simulink model "SistemaPsk"  (R2017a)
settings: Solver=ode45  StartTime=0.0  StopTime=num_bits*tb  RelTol=1e-3
values from neighbouring files (symbols this model uses):
  Amplitud = sqrt(Potencia)    [Parametros_Sistema.m]
  ancho_filtro = rata_bit/2    (= 875)    [Parametros_Sistema.m]
  atenua_voltaje = sqrt(atenua_potencia)    [Parametros_Sistema.m]
  b = tb*0.2    (= 0.000114285714286)    [Parametros_Sistema.m]
  C = 1.5e-9    (= 1.5e-09)    [Parametros_Sistema.m]
  fc = 175e3    (= 175000)    [Parametros_Sistema.m]
  R1 = 200e3    (= 200000)    [Parametros_Sistema.m]
  R2 = 9e3    (= 9000)    [Parametros_Sistema.m]
  rata_bit = 1.75e3    (= 1750)    [Parametros_Sistema.m]
  retardo_canal = long/3e8    [Parametros_Sistema.m]
  retardo_decision = 1/rata_bit    (= 0.000571428571429)    [Parametros_Sistema.m]
  retardo_filtro = 1.7/rata_bit    (= 0.000971428571429)    [Parametros_Sistema.m]
  tb = 1/rb    (= 0.000571428571429)    [Codificacion.m]    (also in Parametros_Sistema.m)
libraries: dsparch4 x5, dspsigops x4, commsynccomp2 x2, powerlib_extras x2, commnoisgen2 x1, commrandsrc3 x1, simulink x1, simulink_extras x1
settings Model: Creator=PROYECTOS_101  LastModifiedBy=PROYECTOS_101

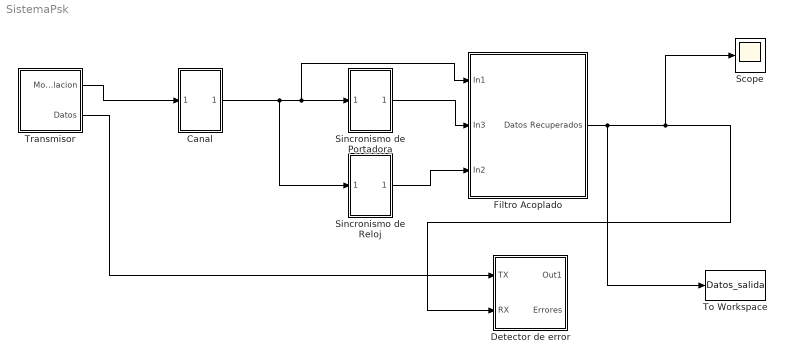
== system SistemaPsk ==
  Canal : Subsystem
  Detector de error : Subsystem
  "Filtro Acoplado " : Subsystem
  Scope : Scope
  Sincronismo de Portadora : Subsystem
  Sincronismo de Reloj : Subsystem
  To Workspace : ToWorkspace  VariableName=Datos_salida  SaveFormat=Structure With Time  SampleTime=-1
      settings: Save2DSignal=2-D array (concatenate along first dimension)
  "Transmisor " : Subsystem
  wires:
  Canal/1(Out1) -> Sincronismo de Reloj/1(In1), "Filtro Acoplado "/1(In1), Sincronismo de Portadora/1(In1)
  Sincronismo de Portadora/1(Out1) -> "Filtro Acoplado "/2(In3)
  Sincronismo de Reloj/1(Out1) -> "Filtro Acoplado "/3(In2)
  "Transmisor "/1(Modulacion) -> Canal/1(In1)
  "Transmisor "/2(Datos) -> Detector de error/1(TX)
  "Filtro Acoplado "/1(Datos Recuperados) -> To Workspace/1, Scope/1, Detector de error/2(RX)

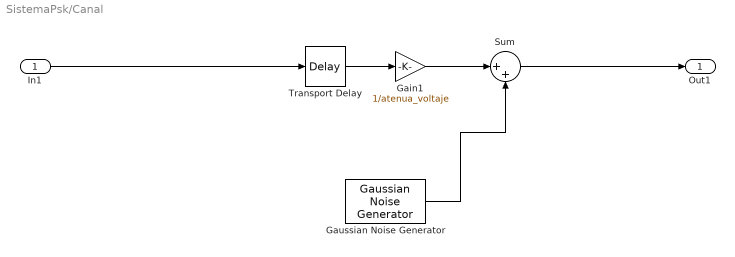
== system SistemaPsk/Canal ==
  In1 : Inport
  Gain1 : Gain  Gain=1/atenua_voltaje
  Gaussian Noise Generator : commnoisgen2/Gaussian Noise Generator  m=0  d=Potencia_ruido  s=61  Ts=1e-8  frameBased=off  sampPerFrame=1  orient=off  outDataType=double
  Sum : Sum  Inputs=|++
  Transport Delay : TransportDelay  DelayTime=retardo_canal
  Out1 : Outport
  wires:
  In1/1 -> Transport Delay/1
  Sum/1 -> Out1/1
  Gaussian Noise Generator/1 -> Sum/2
  Gain1/1 -> Sum/1
  Transport Delay/1 -> Gain1/1

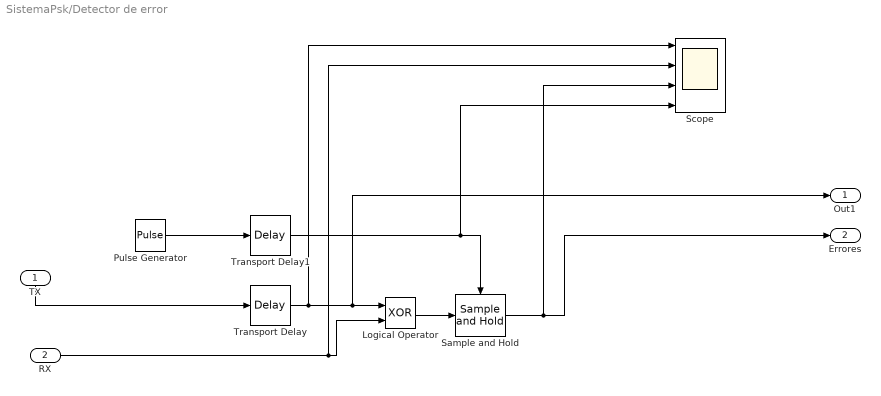
== system SistemaPsk/Detector de error ==
  TX : Inport
  RX : Inport  Port=2
  Logical Operator : Logic  Operator=XOR  AllPortsSameDT=off  OutDataTypeStr=boolean
  Pulse Generator : DiscretePulseGenerator  PulseType=Time based  Period=tb  PulseWidth=50
  Sample and Hold : dspsigops/Sample and Hold  trig=Rising edge  initCond=0  latchinput=off
  Scope : Scope  NumInputPorts=4
  Transport Delay : TransportDelay  DelayTime=retardo_canal+retardo_filtro+retardo_decision
  Transport Delay1 : TransportDelay  DelayTime=retardo_canal+retardo_filtro+retardo_decision
  Out1 : Outport
  Errores : Outport  Port=2
  wires:
  Transport Delay/1 -> Scope/1, Logical Operator/1, Out1/1
  Logical Operator/1 -> Sample and Hold/1
  Pulse Generator/1 -> Transport Delay1/1
  Transport Delay1/1 -> Scope/4, Sample and Hold/Trigger
  Sample and Hold/1 -> Scope/3, Errores/1
  TX/1 -> Transport Delay/1
  RX/1 -> Scope/2, Logical Operator/2

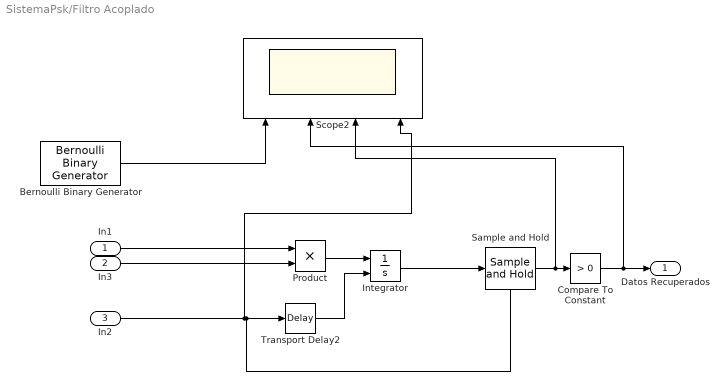
== system SistemaPsk/Filtro Acoplado  ==
  In1 : Inport
  In3 : Inport  Port=2
  In2 : Inport  Port=3
  Bernoulli Binary Generator : commrandsrc3/Bernoulli Binary Generator  ProbabilityOfZero=0.5  SeedSource=Parameter  Seed=61  SampleTime=tb  SamplesPerFrame=1  OutputDataType=double  SimulateUsing=Interpreted execution
  Compare To Constant : simulink/Logic and Bit Operations/Compare To Constant  relop=>  const=0  OutDataTypeStr=boolean
  Integrator : Integrator  ExternalReset=rising
  Product : Product
  Sample and Hold : dspsigops/Sample and Hold  trig=Rising edge  initCond=0  latchinput=off
  Scope2 : Scope  NumInputPorts=4
  Transport Delay2 : TransportDelay  DelayTime=1e-6
  Datos Recuperados : Outport
  wires:
  Integrator/1 -> Sample and Hold/1
  In1/1 -> Product/1
  Sample and Hold/1 -> Scope2/3, Compare To Constant/1
  Product/1 -> Integrator/1
  In2/1 -> Scope2/4, Sample and Hold/Trigger, Transport Delay2/1
  Compare To Constant/1 -> Scope2/2, Datos Recuperados/1
  Transport Delay2/1 -> Integrator/2
  In3/1 -> Product/2
  Bernoulli Binary Generator/1 -> Scope2/1

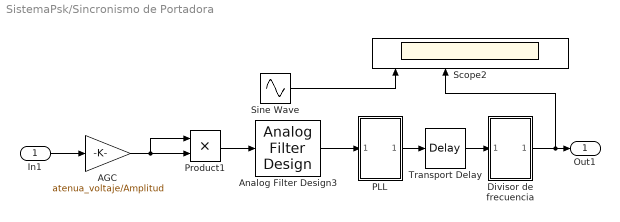
== system SistemaPsk/Sincronismo de Portadora ==
  In1 : Inport
  AGC : Gain  Gain=atenua_voltaje/Amplitud
  Analog Filter Design3 : dsparch4/Analog Filter Design  method=Butterworth  filttype=Bandpass  N=2  Wlo=2*pi*(2*fc-rata_bit)  Whi=2*pi*( 2*fc+rata_bit)  Rp=2  Rs=40
  "Divisor de frecuencia " : Subsystem
  PLL : Subsystem
  Product1 : Product
  Scope2 : Scope  NumInputPorts=4
  Sine Wave : Sin  Amplitude=Amplitud  Frequency=2*pi*(fc)  SampleTime=0
  Transport Delay : TransportDelay  DelayTime=1/(8*fc)
  Out1 : Outport
  wires:
  "Divisor de frecuencia "/1(Out1) -> Scope2/2, Out1/1
  Transport Delay/1 -> "Divisor de frecuencia "/1(In1)
  AGC/1 -> Product1/1, Product1/2
  In1/1 -> AGC/1
  Product1/1 -> Analog Filter Design3/1
  Analog Filter Design3/1 -> PLL/1(In1)
  PLL/1(Out1) -> Transport Delay/1
  Sine Wave/1 -> Scope2/1

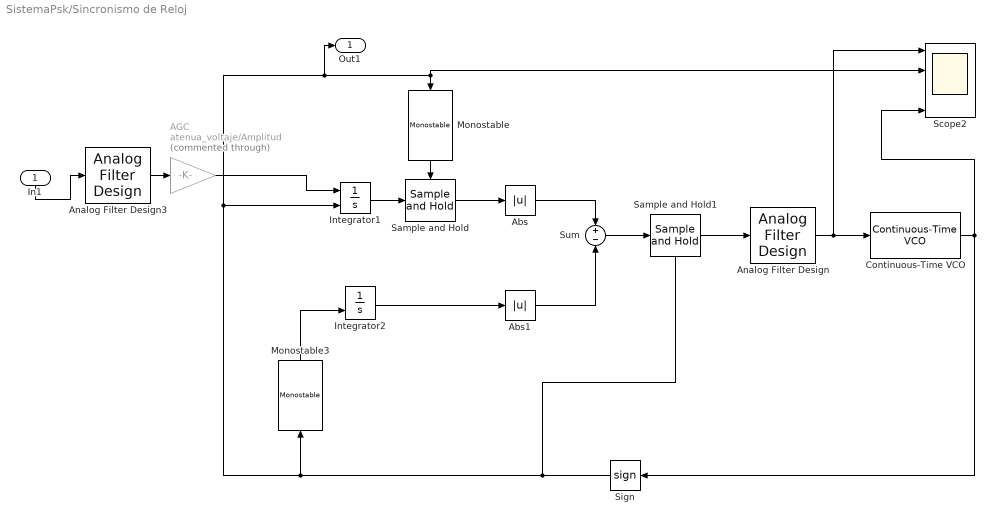
== system SistemaPsk/Sincronismo de Reloj ==
  In1 : Inport
  AGC : Gain  Commented=through  Gain=atenua_voltaje/Amplitud
  Abs : Abs
  Abs1 : Abs
  Analog Filter Design : dsparch4/Analog Filter Design  method=Butterworth  filttype=Lowpass  N=2  Wlo=2*pi*500  Whi=80  Rp=2  Rs=40
  Analog Filter Design3 : dsparch4/Analog Filter Design  method=Butterworth  filttype=Bandpass  N=2  Wlo=2*pi*(fc-rata_bit)  Whi=2*pi*(fc+rata_bit)  Rp=2  Rs=40
  Continuous-Time VCO : commsynccomp2/Continuous-Time VCO  Ac=1  Fc=rata_bit  Kc=1e8  Ph=0
      settings: SourceProductName=Communications System Toolbox  SourceProductBaseCode=CM
  Integrator1 : Integrator  ExternalReset=rising
  Integrator2 : Integrator  ExternalReset=falling
  Monostable : powerlib_extras/Control  Blocks/Monostable  EdgeDetect=Rising  t_mono=tb-b  ic=0
  Monostable3 : powerlib_extras/Control  Blocks/Monostable  EdgeDetect=Rising  t_mono=b  ic=0
  Sample and Hold : dspsigops/Sample and Hold  trig=Falling edge  initCond=0  latchinput=off
  Sample and Hold1 : dspsigops/Sample and Hold  trig=Rising edge  initCond=0  latchinput=off
  Scope2 : Scope  NumInputPorts=4
  Sign : Signum
  Sum : Sum  Inputs=+-
  Out1 : Outport
  wires:
  Abs1/1 -> Sum/2
  Sample and Hold/1 -> Abs/1
  Sum/1 -> Sample and Hold1/1
  Monostable/1 -> Sample and Hold/Trigger
  Sample and Hold1/1 -> Analog Filter Design/1
  Abs/1 -> Sum/1
  Integrator1/1 -> Sample and Hold/1
  Sign/1 -> Sample and Hold1/Trigger, Monostable3/1, Integrator1/2, Out1/1, Scope2/2, Monostable/1
  Integrator2/1 -> Abs1/1
  Monostable3/1 -> Integrator2/2
  Analog Filter Design3/1 -> AGC/1
  In1/1 -> Analog Filter Design3/1
  AGC/1 -> Integrator1/1
  Continuous-Time VCO/1 -> Sign/1, Scope2/4
  Analog Filter Design/1 -> Scope2/1, Continuous-Time VCO/1

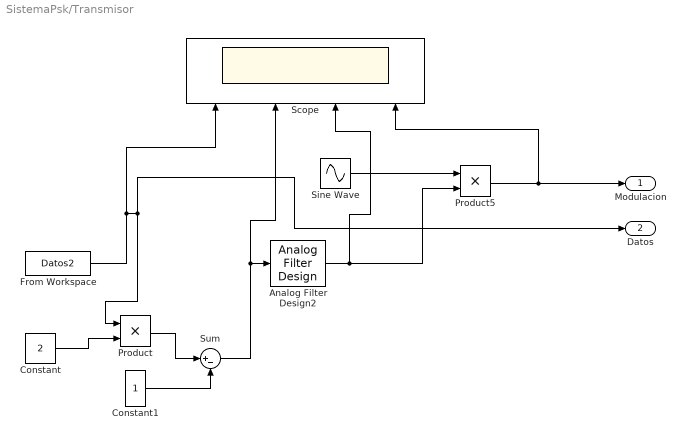
== system SistemaPsk/Transmisor  ==
  Analog Filter Design2 : dsparch4/Analog Filter Design  method=Butterworth  filttype=Lowpass  N=8  Wlo=2*pi*(ancho_filtro)  Whi=2*pi*(800000+90000)  Rp=2  Rs=40
  Constant : Constant  Value=2
  Constant1 : Constant
  From Workspace : FromWorkspace  VariableName=Datos2  SampleTime=0
  Product : Product
  Product5 : Product  RndMeth=Zero
  Scope : Scope  NumInputPorts=4
  Sine Wave : Sin  Amplitude=Amplitud  Frequency=2*pi*(fc)  SampleTime=0
  Sum : Sum  Inputs=|+-
  Modulacion : Outport
  Datos : Outport  Port=2
  wires:
  Analog Filter Design2/1 -> Scope/3, Product5/2
  Sine Wave/1 -> Product5/1
  From Workspace/1 -> Scope/1, Product/1, Datos/1
  Sum/1 -> Scope/2, Analog Filter Design2/1
  Product5/1 -> Scope/4, Modulacion/1
  Product/1 -> Sum/1
  Constant/1 -> Product/2
  Constant1/1 -> Sum/2

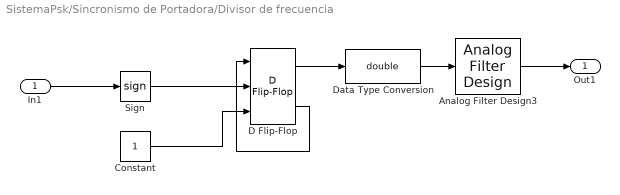
== system SistemaPsk/Sincronismo de Portadora/Divisor de frecuencia  ==
  In1 : Inport
  Analog Filter Design3 : dsparch4/Analog Filter Design  method=Butterworth  filttype=Bandpass  N=2  Wlo=2*pi*(fc-rata_bit)  Whi=2*pi*( fc+rata_bit)  Rp=2  Rs=40
  Constant : Constant
  D Flip-Flop : simulink_extras/Flip Flops/D Flip-Flop
      settings: SourceProductName=Simulink
  Data Type Conversion : DataTypeConversion  OutDataTypeStr=double
  Sign : Signum
  Out1 : Outport
  wires:
  Analog Filter Design3/1 -> Out1/1
  Sign/1 -> D Flip-Flop/2
  Constant/1 -> D Flip-Flop/3
  D Flip-Flop/2 -> D Flip-Flop/1
  In1/1 -> Sign/1
  Data Type Conversion/1 -> Analog Filter Design3/1
  D Flip-Flop/1 -> Data Type Conversion/1

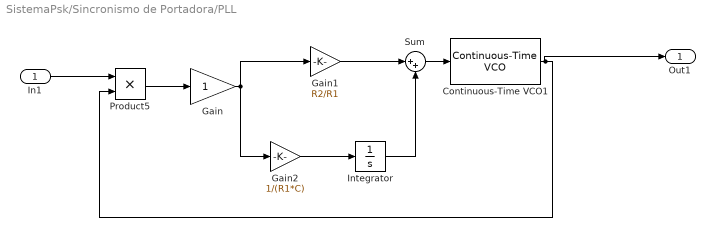
== system SistemaPsk/Sincronismo de Portadora/PLL ==
  In1 : Inport
  Continuous-Time VCO1 : commsynccomp2/Continuous-Time VCO  Ac=1  Fc=2*(fc)  Kc=1e6  Ph=0
      settings: SourceProductName=Communications System Toolbox  SourceProductBaseCode=CM
  Gain : Gain
  Gain1 : Gain  Gain=R2/R1
  Gain2 : Gain  Gain=1/(R1*C)
  Integrator : Integrator
  Product5 : Product
  Sum : Sum  Inputs=|++
  Out1 : Outport
  wires:
  Gain1/1 -> Sum/1
  Gain/1 -> Gain2/1, Gain1/1
  Continuous-Time VCO1/1 -> Out1/1, Product5/2
  Sum/1 -> Continuous-Time VCO1/1
  Gain2/1 -> Integrator/1
  Product5/1 -> Gain/1
  Integrator/1 -> Sum/2
  In1/1 -> Product5/1
